simulink subsystem "torque_decompose_sub"  (R2025b)
settings: Solver=VariableStepAuto  StartTime=0.0  StopTime=10.0  RelTol=1e-3
settings Model: Creator=lew11  LastModifiedBy=lew11

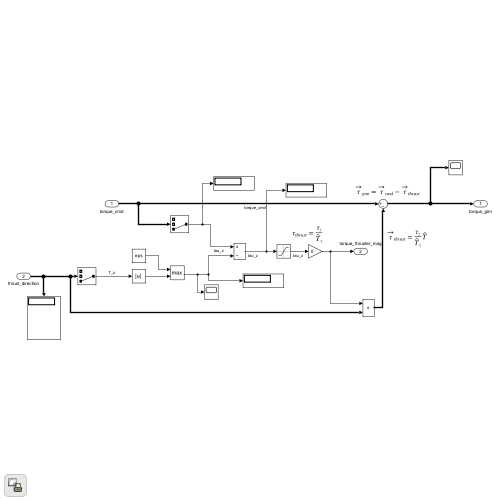
[thumbnail: Simulink's stored preview of the top-level diagram]
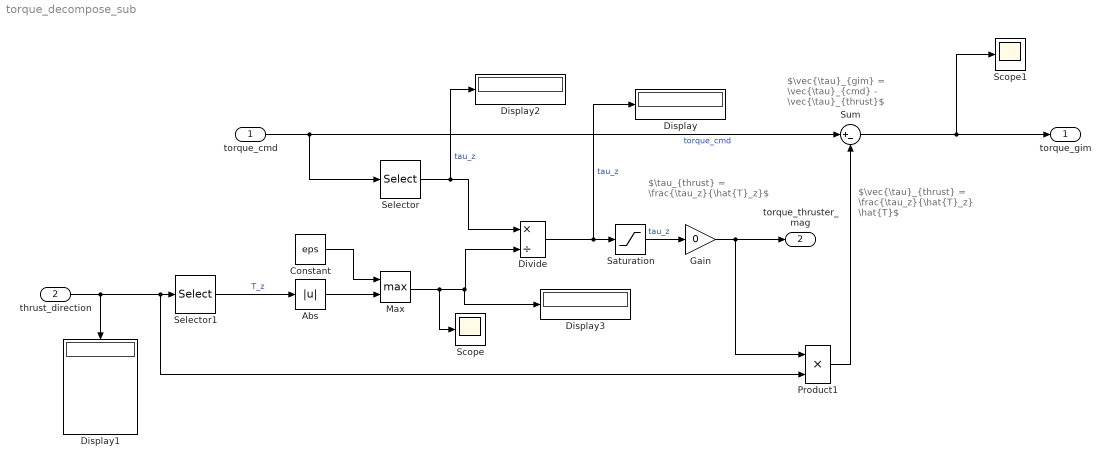
== system torque_decompose_sub ==
  note: $\vec{\tau}_{thrust} = \frac{\tau_z}{\hat{T}_z} \hat{T}$
  note: $\vec{\tau}_{gim} = \vec{\tau}_{cmd} - \vec{\tau}_{thrust}$
  note: $\tau_{thrust} = \frac{\tau_z}{\hat{T}_z}$
  torque_cmd : Inport  PortDimensions=3
  thrust_direction : Inport  Port=2  PortDimensions=3
  Abs : Abs  SaturateOnIntegerOverflow=off
  Constant : Constant  Value=eps
  Display{,1..3} (4 alike) : Display
  Divide : Product  Inputs=*/
  Gain : Gain  Gain=0
  Max : MinMax  Function=max  Inputs=2
  Product1 : Product
  Saturation : Saturate  UpperLimit=.2  LowerLimit=-.2
  Scope : Scope
      settings: ActiveDisplayYMinimum=-1  ActiveDisplayYMaximum=1  DataLoggingVariableName=ScopeData9
  Scope1 : Scope
      settings: ActiveDisplayYMinimum=-30.146084851817548  ActiveDisplayYMaximum=35.066245942464121  DataLoggingVariableName=ScopeData10
  Selector : Selector  InputPortWidth=3  IndexOptions=Index vector (dialog)  Indices=3  OutputSizes=1
  Selector1 : Selector  InputPortWidth=3  IndexOptions=Index vector (dialog)  Indices=3  OutputSizes=1
  Sum : Sum  Inputs=|+-
  torque_gim : Outport  PortDimensions=3
  torque_thruster_mag : Outport  Port=2  PortDimensions=1
  wires:
  Saturation/1 -> Gain/1  "tau_z"
  Selector1/1 -> Abs/1  "T_z"
  torque_cmd/1 -> Sum/1, Selector/1  "torque_cmd"
  Divide/1 -> Display/1, Saturation/1  "tau_z"
  Sum/1 -> torque_gim/1, Scope1/1
  Constant/1 -> Max/1
  Product1/1 -> Sum/2
  thrust_direction/1 -> Product1/2, Selector1/1, Display1/1
  Selector/1 -> Display2/1, Divide/1  "tau_z"
  Abs/1 -> Max/2
  Max/1 -> Divide/2, Display3/1, Scope/1
  Gain/1 -> torque_thruster_mag/1, Product1/1
